simulink model "ControleNL_Degrau"  (R2020b)
settings: Solver=FixedStepAuto  StartTime=0  StopTime=10  FixedStep=1e-3  RelTol=1e-3
values from neighbouring files (symbols this model uses):
  alpha = 1.25    [kermani_parameters.m]    (also in teste_controle_nao_linear.m)
  Beff = 50    [kermani_parameters.m]    (also in teste_controle_nao_linear.m)
  Fc = phi*Beff    (= 2173.5)    [kermani_parameters.m]    (also in teste_controle_nao_linear.m)
  freq = 0.1    [kermani_parameters.m]    (also in teste_controle_nao_linear.m)
  Fs = (phi+10)*Beff    (= 2673.5)    [kermani_parameters.m]    (also in teste_controle_nao_linear.m)
  Jeff = 0.5    [kermani_parameters.m]    (also in teste_controle_nao_linear.m)
  K = Km/(R*Beff)    (= 40)    [kermani_parameters.m]    (also in teste_controle_nao_linear.m = 0.785398163397)
  K_NL = Km_NL/(R*Beff)    (= 48.694)    [kermani_parameters.m]    (also in teste_controle_nao_linear.m)
  r = 1./[231.22*4 139.138 139.138 231.22 231.22]    [kermani_parameters.m]    (also in teste_controle_nao_linear.m)
  sigma0 = 200*Beff    (= 10000)    [kermani_parameters.m]    (also in teste_controle_nao_linear.m)
  sigma1 = 20*Beff    (= 1000)    [kermani_parameters.m]    (also in teste_controle_nao_linear.m)
  sigma2 = 0.2*Beff    (= 10)    [kermani_parameters.m]    (also in teste_controle_nao_linear.m)
libraries: simulink_extras x3
(part 5 of 5)

== matlab function ControleNL_Degrau/Dinâmica do robô não linear/Perturbação/MATLAB Function3 ==
  data: M input; V input; tau1 output; G input; ddTh input
function tau1  = calcul_dk1(M, V, G, ddTh)

tau1 = M(1,2)*ddTh(2) + M(1,3)*ddTh(3) + M(1,4)*ddTh(4) + M(1,5)*ddTh(5) ...
       + V(1) + G(1);
